simulink model "sfun_demo_sin"  (R2018b)
settings: Solver=VariableStepAuto  StartTime=0.0  StopTime=10.0  RelTol=1e-3
settings Model: Creator=Shun  LastModifiedBy=Shun

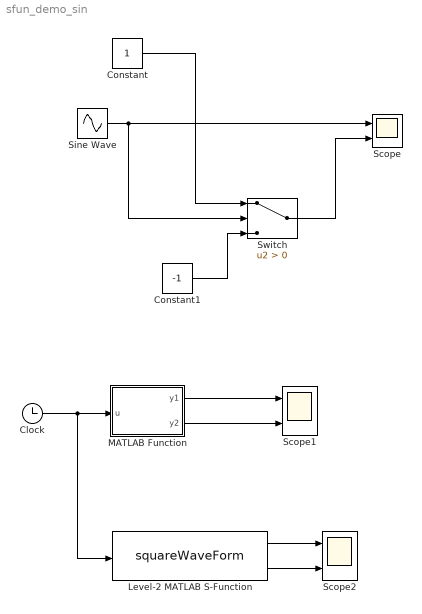
== system sfun_demo_sin ==
  Clock : Clock
  Constant : Constant
  Constant1 : Constant  Value=-1
  Level-2 MATLAB S-Function : M-S-Function  FunctionName=squareWaveForm
  MATLAB Function : MATLAB Function  TreatAsAtomicUnit=on
  Scope : Scope  NumInputPorts=2
  Scope1 : Scope  NumInputPorts=2
  Scope2 : Scope  NumInputPorts=2
  Sine Wave : Sin  SampleTime=0
  Switch : Switch  Criteria=u2 > Threshold
  wires:
  Sine Wave/1 -> Switch/2, Scope/1
  Constant/1 -> Switch/1
  Constant1/1 -> Switch/3
  Switch/1 -> Scope/2
  MATLAB Function/1(y1) -> Scope1/1
  MATLAB Function/2(y2) -> Scope1/2
  Clock/1 -> Level-2 MATLAB S-Function/1, MATLAB Function/1(u)
  Level-2 MATLAB S-Function/1 -> Scope2/1
  Level-2 MATLAB S-Function/2 -> Scope2/2

== matlab function sfun_demo_sin/MATLAB Function ==
  data: u input; y1 output; y2 output
function [y1,y2] = fcn(u)

y1 = sin(u);
if y1 >0
    y2=1;
else
    y2 = -1;
end
end
